simulink model "sampleModel446"  (R2021b)
settings: Solver=VariableStepAuto  StartTime=0.0  StopTime=10.0  RelTol=1e-3
undefined symbols (not defined in the file): Newton, Raphson
libraries: simulink x5, slpidlib x1
settings Model: Creator=cemery  LastModifiedBy=cemery
settings SolverCC: AlgebraicLoopSolver=TrustRegion
settings DataIOCC: ReturnWorkspaceOutputs=off
settings DebuggingCC: SFMachineParentedDataDiag=warning  ArithmeticOperatorsInVariantConditions=warning
settings SFSimCC: SimUseLocalCustomCode=off  CustomCodeUndefinedFunction=UseInterfaceOnly
settings RTWCC: RTWUseLocalCustomCode=off

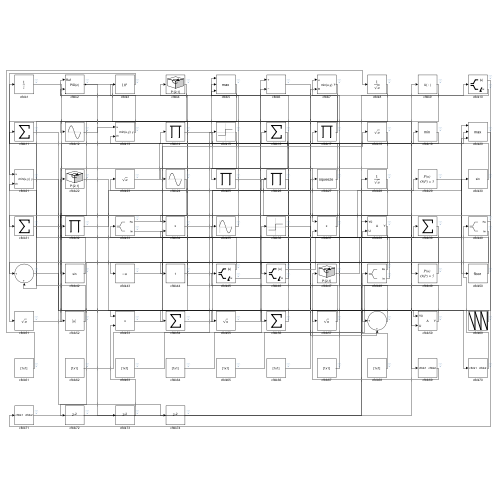
[thumbnail: Simulink's stored preview of the top-level diagram]
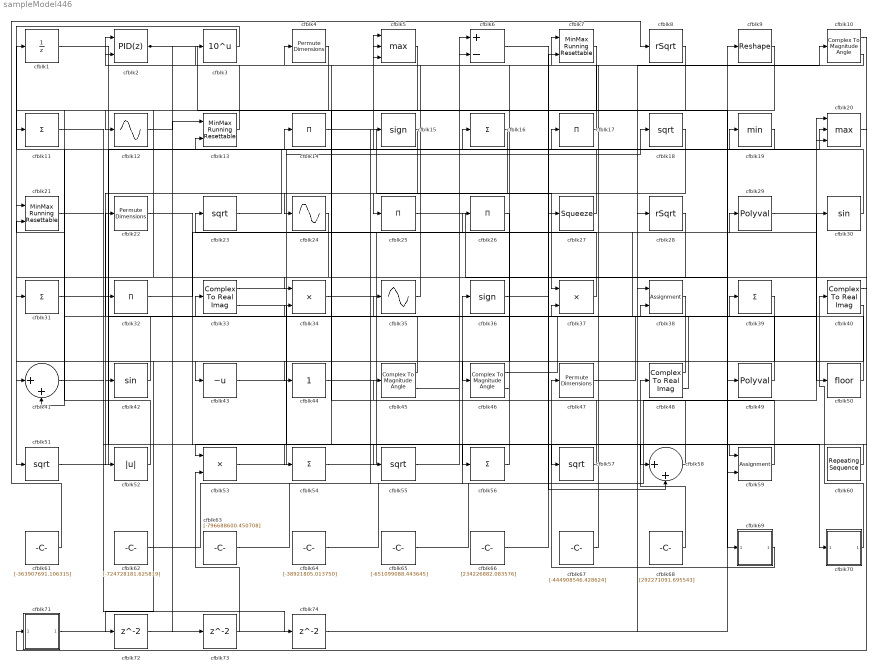
== system sampleModel446 ==
  cfblk1 : UnitDelay  HasFrameUpgradeWarning=on
  cfblk10 : ComplexToMagnitudeAngle
  cfblk{11,16,31,39,54,56} (6 alike) : Sum  Inputs=+
  cfblk12 : Sin  TimeSource=Use external signal  SampleTime=0
  cfblk13 : simulink/Math Operations/MinMax Running Resettable  Function=min  vinit=0.0
  cfblk{14,17,25..26,32} (5 alike) : Product  Inputs=*
  cfblk15 : Signum
  cfblk{18,23,51,55,57} (5 alike) : Sqrt  SaturateOnIntegerOverflow=on
  cfblk19 : MinMax
  cfblk2 : slpidlib/PID Controller (2DOF)  Controller=PID  Form=Parallel  TimeDomain=Discrete-time  UseExternalTs=off  SampleTime=1  IntegratorMethod=Forward Euler  FilterMethod=Forward Euler  ControllerParametersSource=internal  P=1  I=1  D=0  UseFilter=on  N=100  b=1  c=1  TunerSelectOption=Transfer Function Based (PID Tuner App)  InitialConditionSource=internal  InitialConditionForIntegrator=0  InitialConditionForFilter=0  DifferentiatorICPrevScaledInput=0  ExternalReset=none  TrackingMode=off  Kt=1  LimitOutput=off  SatLimitsSource=internal  UpperSaturationLimit=inf  LowerSaturationLimit=-inf  LinearizeAsGain=off  AntiWindupMode=none  Kb=1  POutMin=[]  POutMax=[]  IOutMin=[]  IOutMax=[]  DOutMin=[]  DOutMax=[]  NOutMin=[]  NOutMax=[]  bOutMin=[]  bOutMax=[]  cOutMin=[]  cOutMax=[]  SumOutMin=[]  SumOutMax=[]  SaturationOutMin=[]  SaturationOutMax=[]  PParamMin=[]  PParamMax=[]  IParamMin=[]  IParamMax=[]  DParamMin=[]  DParamMax=[]  NParamMin=[]  NParamMax=[]  bParamMin=[]  bParamMax=[]  cParamMin=[]  cParamMax=[]  KbParamMin=[]  KbParamMax=[]  KtParamMin=[]  KtParamMax=[]  KbOutMin=[]  KbOutMax=[]  KtOutMin=[]  KtOutMax=[]  IntegratorOutMin=[]  IntegratorOutMax=[]  FilterOutMin=[]  FilterOutMax=[]  SumI1OutMin=[]  SumI1OutMax=[]  SumI2OutMin=[]  SumI2OutMax=[]  SumI3OutMin=[]  SumI3OutMax=[]  SumI4OutMin=[]  SumI4OutMax=[]  SumDOutMin=[]  SumDOutMax=[]  Sum1OutMin=[]  Sum1OutMax=[]  Sum2OutMin=[]  Sum2OutMax=[]  Sum3OutMin=[]  Sum3OutMax=[]  DifferentiatorOutMin=[]  DifferentiatorOutMax=[]  FilterDiffOutCoefMin=[]  FilterDiffOutCoefMax=[]  ReciprocalOutMin=[]  ReciprocalOutMax=[]  SumDenOutMin=[]  SumDenOutMax=[]  SumNumOutMin=[]  SumNumOutMax=[]  DivideOutMin=[]  DivideOutMax=[]  UdiffTsProdOutMin=[]  UdiffTsProdOutMax=[]  NTsProdOutMin=[]  NTsProdOutMax=[]  UintegralTsProdOutMin=[]  UintegralTsProdOutMax=[]  UngainTsProdOutMin=[]  UngainTsProdOutMax=[]  IntegratorContinuousStateAttributes=''  IntegratorStateMustResolveToSignalObject=off  IntegratorRTWStateStorageClass=Auto  FilterContinuousStateAttributes=''  FilterStateMustResolveToSignalObject=off  FilterRTWStateStorageClass=Auto  ParallelPVariant=InternalParameters  IdealPVariant=Disabled  IVariant=InternalParameters  DVariant=InternalParameters  bVariant=InternalParameters  cVariant=InternalParameters  IntegratorVariant=Discrete  SatVariant=Disabled  AWVariant=Passthrough  PCopyVariant=Disabled  TRVariant=Disabled  FdbkBlocksVariant=Forward  IdealPFdbkVariant=Disabled  SatFdbkVariant=Disabled  DerivativeFilterVariant=ForwardEulerFilter  NVariant=InternalParameters  NCopyVariant=Disabled  FilterICVariant=InternalICsFilter  IntegratorICVariant=InternalICs  ExternalResetVariant=Disabled  TRSumVariant=Passthrough  SumFdbkVariant=Disabled  SumVariant=Sum_PID  TsampFilterVariant=InternalTs  TsampNgainVariant=Passthrough  TsampIntegralVariant=Passthrough  ExternalSaturationOutDataTypeStr=Inherit: Same as second input
      settings: SourceProductBaseCode=SL
  cfblk20 : MinMax  Function=max  Inputs=3
  cfblk21 : simulink/Math Operations/MinMax Running Resettable  Function=min  vinit=0.0
  cfblk22 : PermuteDimensions
  cfblk24 : Sin  TimeSource=Use external signal  SampleTime=0
  cfblk27 : Squeeze
  cfblk28 : Sqrt  Operator=rSqrt  AlgorithmType=Newton-Raphson  SaturateOnIntegerOverflow=on
  cfblk29 : Polyval  Coefs=[ +2.081618890e-019, -1.441693666e-014, +4.719686976e-010, -8.536869453e-006, +1.621573104e-001, -8.087801117e+001 ]
  cfblk3 : Math  Operator=10^u  SignedPower=on  SaturateOnIntegerOverflow=on
  cfblk30 : Trigonometry
  cfblk33 : ComplexToRealImag
  cfblk34 : Product
  cfblk35 : Sin  TimeSource=Use external signal  SampleTime=0
  cfblk36 : Signum
  cfblk37 : Product  Inputs=**
  cfblk38 : Assignment  DiagnosticForDimensions=Warning  IndexOptions=Index vector (dialog)  Indices=1  OutputSizes=1
  cfblk4 : PermuteDimensions
  cfblk40 : ComplexToRealImag
  cfblk41 : Sum  Inputs=|++
  cfblk42 : Trigonometry
  cfblk43 : UnaryMinus
  cfblk44 : simulink/Math Operations/Slider Gain  gain=1  low=0  high=2
  cfblk45 : ComplexToMagnitudeAngle
  cfblk46 : ComplexToMagnitudeAngle
  cfblk47 : PermuteDimensions
  cfblk48 : ComplexToRealImag
  cfblk49 : Polyval  Coefs=[ +2.081618890e-019, -1.441693666e-014, +4.719686976e-010, -8.536869453e-006, +1.621573104e-001, -8.087801117e+001 ]
  cfblk5 : MinMax  Function=max  Inputs=3
  cfblk50 : Rounding
  cfblk52 : Abs
  cfblk53 : Product
  cfblk58 : Sum  Inputs=|++
  cfblk59 : Assignment  DiagnosticForDimensions=Warning  IndexOptions=Index vector (dialog)  Indices=1  OutputSizes=1
  cfblk6 : Sum  Inputs=+-
  cfblk60 : simulink/Sources/Repeating Sequence  rep_seq_t=[0 2]  rep_seq_y=[361758383.384675, -700642344.613808]
  cfblk61 : Constant  Value=[-363907691.106315]  SampleTime=1
  cfblk62 : Constant  Value=[-724728181.625819]  SampleTime=1
  cfblk63 : Constant  Value=[-796688600.450708]  SampleTime=1
  cfblk64 : Constant  Value=[-38921805.013750]  SampleTime=1
  cfblk65 : Constant  Value=[-651099088.443645]  SampleTime=1
  cfblk66 : Constant  Value=[234226882.083576]  SampleTime=1
  cfblk67 : Constant  Value=[-444908546.428624]  SampleTime=1
  cfblk68 : Constant  Value=[292271091.695543]  SampleTime=1
  cfblk69 : Subsystem
  cfblk7 : simulink/Math Operations/MinMax Running Resettable  Function=min  vinit=0.0
  cfblk70 : Subsystem
  cfblk71 : Subsystem
  cfblk72 : Delay  SampleTime=1
  cfblk73 : Delay  SampleTime=1
  cfblk74 : Delay  SampleTime=1
  cfblk8 : Sqrt  Operator=rSqrt  AlgorithmType=Newton-Raphson  SaturateOnIntegerOverflow=on
  cfblk9 : Reshape
  wires:
  cfblk68/1 -> cfblk48/1
  cfblk51/1 -> cfblk14/1
  cfblk33/1 -> cfblk18/1
  cfblk47/1 -> cfblk39/1
  cfblk69/1(cfblk2) -> cfblk47/1
  cfblk18/1 -> cfblk25/1
  cfblk16/1 -> cfblk52/1
  cfblk46/1 -> cfblk29/1
  cfblk3/1 -> cfblk51/1
  cfblk27/1 -> cfblk1/1
  cfblk14/1 -> cfblk37/1
  cfblk66/1 -> cfblk27/1
  cfblk17/1 -> cfblk2/1
  cfblk38/1 -> cfblk43/1
  cfblk1/1 -> cfblk70/1(cfblk1)
  cfblk43/1 -> cfblk19/1
  cfblk12/1 -> cfblk13/1
  cfblk61/1 -> cfblk8/1
  cfblk64/1 -> cfblk36/1
  cfblk37/1 -> cfblk23/1
  cfblk71/1(cfblk2) -> cfblk28/1
  cfblk25/1 -> cfblk49/1
  cfblk70/1(cfblk2) -> cfblk40/1
  cfblk50/1 -> cfblk22/1
  cfblk63/1 -> cfblk30/1
  cfblk20/1 -> cfblk71/1(cfblk1)
  cfblk15/1 -> cfblk24/1
  cfblk19/1 -> cfblk13/2
  cfblk45/1 -> cfblk33/1
  cfblk9/1 -> cfblk21/1
  cfblk59/1 -> cfblk7/1
  cfblk52/1 -> cfblk11/1
  cfblk33/2 -> cfblk56/1
  cfblk56/1 -> cfblk16/1
  cfblk2/1 -> cfblk69/1(cfblk1), cfblk73/1
  cfblk24/1 -> cfblk42/1
  cfblk48/1 -> cfblk41/1
  cfblk34/1 -> cfblk7/2
  cfblk54/1 -> cfblk20/1
  cfblk48/2 -> cfblk37/2
  cfblk28/1 -> cfblk31/1
  cfblk49/1 -> cfblk4/1
  cfblk32/1 -> cfblk26/1
  cfblk8/1 -> cfblk41/2
  cfblk41/1 -> cfblk59/1
  cfblk30/1 -> cfblk5/1
  cfblk67/1 -> cfblk17/1
  cfblk23/1 -> cfblk20/2
  cfblk10/1 -> cfblk34/1
  cfblk55/1 -> cfblk6/1
  cfblk53/1 -> cfblk35/1
  cfblk46/2 -> cfblk5/2
  cfblk31/1 -> cfblk38/2
  cfblk5/1 -> cfblk54/1
  cfblk4/1 -> cfblk32/1
  cfblk40/1 -> cfblk53/1
  cfblk22/1 -> cfblk58/1
  cfblk29/1 -> cfblk50/1
  cfblk26/1 -> cfblk46/1
  cfblk36/1 -> cfblk59/2
  cfblk45/2 -> cfblk6/2
  cfblk44/1 -> cfblk20/3
  cfblk60/1 -> cfblk57/1
  cfblk35/1 -> cfblk5/3
  cfblk10/2 -> cfblk3/1
  cfblk7/1 -> cfblk12/1
  cfblk62/1 -> cfblk15/1
  cfblk57/1 -> cfblk45/1
  cfblk40/2 -> cfblk44/1
  cfblk11/1 -> cfblk55/1
  cfblk13/1 -> cfblk2/2
  cfblk6/1 -> cfblk58/2
  cfblk58/1 -> cfblk34/2
  cfblk42/1 -> cfblk21/2
  cfblk65/1 -> cfblk10/1
  cfblk39/1 -> cfblk72/1
  cfblk72/1 -> cfblk38/1
  cfblk73/1 -> cfblk53/2
  cfblk21/1 -> cfblk74/1
  cfblk74/1 -> cfblk9/1

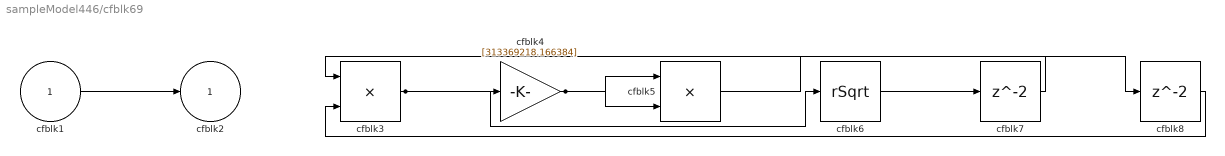
== system sampleModel446/cfblk69 ==
  cfblk1 : Inport
  cfblk3 : Product
  cfblk4 : Gain  Gain=[313369218.166384]
  cfblk5 : Product  Inputs=**
  cfblk6 : Sqrt  Operator=rSqrt  AlgorithmType=Newton-Raphson  SaturateOnIntegerOverflow=on
  cfblk7 : Delay  SampleTime=1
  cfblk8 : Delay  SampleTime=1
  cfblk2 : Outport  VectorParamsAs1DForOutWhenUnconnected=off
  wires:
  cfblk1/1 -> cfblk2/1
  cfblk4/1 -> cfblk5/1, cfblk5/2
  cfblk3/1 -> cfblk6/1, cfblk4/1
  cfblk6/1 -> cfblk7/1
  cfblk7/1 -> cfblk3/1
  cfblk5/1 -> cfblk8/1
  cfblk8/1 -> cfblk3/2

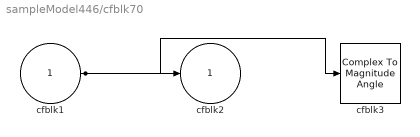
== system sampleModel446/cfblk70 ==
  cfblk1 : Inport
  cfblk3 : ComplexToMagnitudeAngle
  cfblk2 : Outport  VectorParamsAs1DForOutWhenUnconnected=off
  wires:
  cfblk1/1 -> cfblk2/1, cfblk3/1

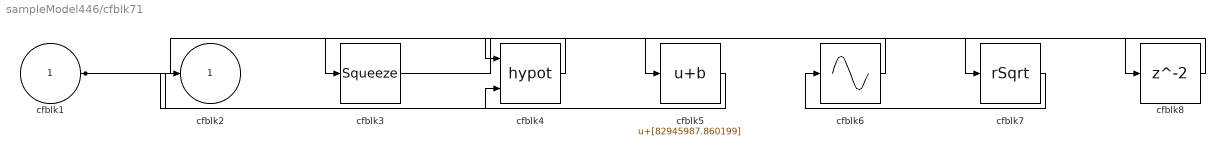
== system sampleModel446/cfblk71 ==
  cfblk1 : Inport
  cfblk3 : Squeeze
  cfblk4 : Math  Operator=hypot  SignedPower=on  SaturateOnIntegerOverflow=on
  cfblk5 : Bias  Bias=[82945987.860199]
  cfblk6 : Sin  TimeSource=Use external signal  SampleTime=0
  cfblk7 : Sqrt  Operator=rSqrt  AlgorithmType=Newton-Raphson  SaturateOnIntegerOverflow=on
  cfblk8 : Delay  SampleTime=1
  cfblk2 : Outport  VectorParamsAs1DForOutWhenUnconnected=off
  wires:
  cfblk1/1 -> cfblk7/1, cfblk4/2
  cfblk7/1 -> cfblk6/1
  cfblk5/1 -> cfblk2/1
  cfblk6/1 -> cfblk5/1
  cfblk4/1 -> cfblk3/1
  cfblk3/1 -> cfblk8/1
  cfblk8/1 -> cfblk4/1
